simulink model "acc"  (Simulink 7.3)
settings: Solver=ode45  StartTime=0.0  StopTime=1000  RelTol=1e-3
libraries: xbsIndex_r4 x26, xps_library x4, casper_library x4
settings Model: Creator=rprimian  LastModifiedBy=rprimian

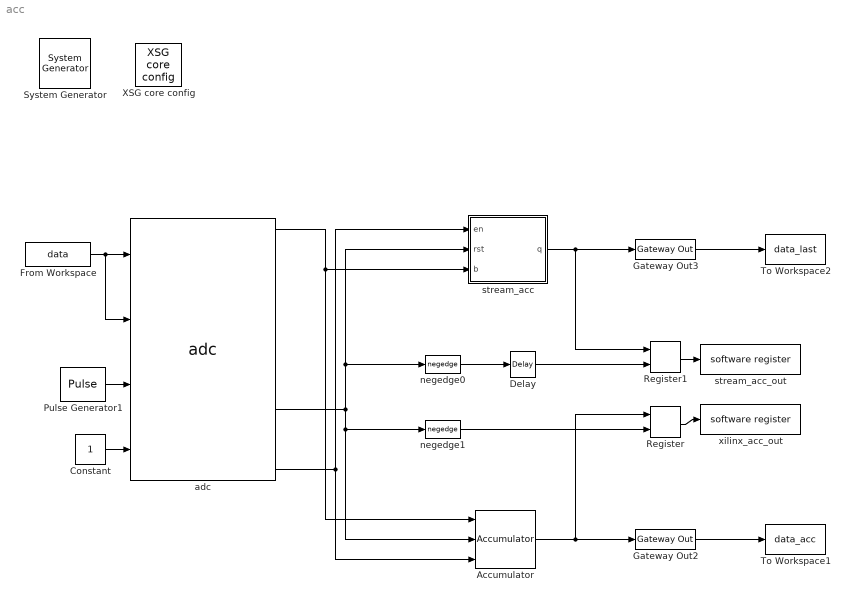
== system acc ==
  " System Generator" : xbsIndex_r4/ System Generator  Tag=genX  SystemSampleTime=-1  xilinxfamily=virtex5  part=xc5vsx95t  speed=-1  package=ff1136  synthesis_tool=XST  clock_wrapper=Clock Enables  directory=./acc/sysgen  testbench=off  simulink_period=1  sysclk_period=3.9062  dcm_input_clock_period=100  incr_netlist=off  trim_vbits=Everywhere in SubSystem  dbl_ovrd=According to Block Masks  core_generation=According to Block Masks  run_coregen=off  deprecated_control=off  eval_field=0  block_type=sysgen
      settings: block_version=11.3
  Accumulator : xbsIndex_r4/Accumulator  operation=Add  n_bits=32  overflow=Flag as error  scale=1  rst=on  hasbypass=off  en=on  dbl_ovrd=off  use_behavioral_HDL=on  implementation=Fabric  block_type=accum
      settings: block_version=11.3
  Constant : Constant  OutDataType=fixdt(1, 16)  OutScaling=2^0
  Delay : xbsIndex_r4/Delay  en=off  latency=7  dbl_ovrd=off  reg_retiming=off  block_type=delay
      settings: block_version=11.3
  From Workspace : FromWorkspace  VariableName=data  SampleTime=0.25  Interpolate=off  OutputAfterFinalValue=Setting to zero
  Gateway Out2 : xbsIndex_r4/Gateway Out  hdl_port=on  timing_constraint=None  locs_specified=off  LOCs={}  block_type=gatewayout
      settings: infoedit="Gateway out block.  Converts Xilinx fixed point inputs into ouputs of type Simulink integer, double, or fixed point.<br><br>Hardware notes:  In hardware these blocks become top level output ports or are discarded, depending on how they are configured."  block_version=11.3
  Gateway Out3 : xbsIndex_r4/Gateway Out  hdl_port=on  timing_constraint=None  locs_specified=off  LOCs={}  block_type=gatewayout
      settings: infoedit="Gateway out block.  Converts Xilinx fixed point inputs into ouputs of type Simulink integer, double, or fixed point.<br><br>Hardware notes:  In hardware these blocks become top level output ports or are discarded, depending on how they are configured."  block_version=11.3
  Pulse Generator1 : DiscretePulseGenerator  Amplitude=1  Period=100  PulseWidth=1  PhaseDelay=50-7  SampleTime=1
  Register : xbsIndex_r4/Register  init=0  rst=off  en=on  dbl_ovrd=off  block_type=register
      settings: block_version=11.3
  Register1 : xbsIndex_r4/Register  init=0  rst=off  en=on  dbl_ovrd=off  block_type=register
      settings: block_version=11.3
  To Workspace1 : ToWorkspace  VariableName=data_acc  SampleTime=-1  SaveFormat=Array
  To Workspace2 : ToWorkspace  VariableName=data_last  SampleTime=-1  SaveFormat=Array
  XSG core config : xps_library/XSG core config  Tag=xps:xsg  SystemSampleTime=-1  hw_sys=ROACH:sx95t  ibob_linux=off  clk_src=adc0_clk  iBOB_clk_src=sys_clk  BEE2_ctrl_clk_src=sys_clk  BEE2_usr_clk_src=sys_clk  ROACH_clk_src=adc0_clk  CORR_clk_src=sys_clk  gpio_clk_io_group=iBOB:sma  gpio_clk_bit_index=0  clk_rate=256  sample_period=1  synthesis_tool=XST  mpc_type=powerpc440_ext
  adc : xps_library/adc  Tag=xps:adc  SystemSampleTime=-1  adc_brd=adc0  adc_clk_rate=1024  adc_interleave=off  sample_period=1
  negedge0 : casper_library/Misc/negedge  Tag=Rising Edge Detector  SystemSampleTime=-1
  negedge1 : casper_library/Misc/negedge  Tag=Rising Edge Detector  SystemSampleTime=-1
  stream_acc : Subsystem  mask{data_type=Signed, bits=32, bin_pt=14, add_latency=2}
      mask prompts: data_type "Output Data Type"; bits "Output Bit Width:"; bin_pt "Output Binary Point:"; add_latency "Adder Latency"
      mask StyleString: popup(Signed|Unsigned),edit,edit,edit
  stream_acc_out : xps_library/software register  Tag=xps:sw_reg  SystemSampleTime=-1  io_dir=To Processor  arith_type=Unsigned  bitwidth=32  bin_pt=0  sample_period=1  gw_name=acc_stream_acc_out_user_data_in
  xilinx_acc_out : xps_library/software register  Tag=xps:sw_reg  SystemSampleTime=-1  io_dir=To Processor  arith_type=Unsigned  bitwidth=32  bin_pt=0  sample_period=1  gw_name=acc_xilinx_acc_out_user_data_in
  wires:
  adc/1 -> Accumulator/1, stream_acc/3(b)
  Accumulator/1 -> Gateway Out2/1, Register/1
  Gateway Out2/1 -> To Workspace1/1
  Gateway Out3/1 -> To Workspace2/1
  stream_acc/1(q) -> Gateway Out3/1, Register1/1
  adc/17 -> stream_acc/1(en), Accumulator/3
  adc/13 -> stream_acc/2(rst), negedge0/1, Accumulator/2, negedge1/1
  From Workspace/1 -> adc/1, adc/2
  Pulse Generator1/1 -> adc/3
  Constant/1 -> adc/4
  Register1/1 -> stream_acc_out/1
  Register/1 -> xilinx_acc_out/1
  negedge0/1 -> Delay/1
  negedge1/1 -> Register/2
  Delay/1 -> Register1/2

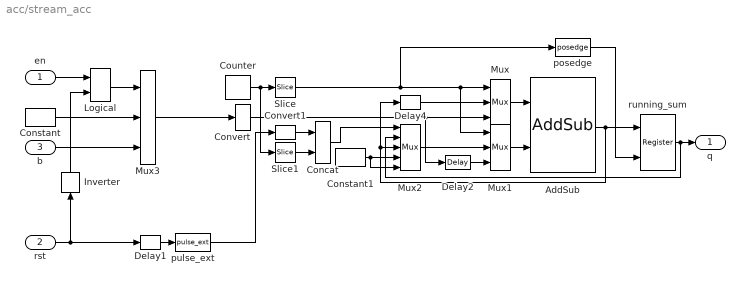
== system acc/stream_acc ==
  en : Inport
  rst : Inport  Port=2
  b : Inport  Port=3
  AddSub : xbsIndex_r4/AddSub  mode=Addition  use_carryin=off  use_carryout=off  en=off  latency=add_latency  precision=User Defined  arith_type="Signed  (2's comp)"  n_bits=32  bin_pt=14  quantization=Truncate  overflow=Flag as error  dbl_ovrd=off  use_behavioral_HDL=off  hw_selection=Fabric  pipelined=off  block_type=addsub
      settings: block_version=11.3
  Concat : xbsIndex_r4/Concat  num_inputs=2  dbl_ovrd=off  block_type=concat
      settings: block_version=11.3
  Constant : xbsIndex_r4/Constant  arith_type=Signed (2's comp)  const=0  n_bits=16  bin_pt=14  explicit_period=on  period=1  equ=P=C  opselect=C  inp2=PCIN>>17  opr=+  inp1=P  carry=CIN  dbl_ovrd=off  block_type=constant
      settings: block_version=11.3
  Constant1 : xbsIndex_r4/Constant  arith_type=Signed (2's comp)  const=0  n_bits=32  bin_pt=14  explicit_period=on  period=1  equ=P=C  opselect=C  inp2=PCIN>>17  opr=+  inp1=P  carry=CIN  dbl_ovrd=off  block_type=constant
      settings: block_version=11.3
  Convert : xbsIndex_r4/Convert  arith_type="Signed  (2's comp)"  n_bits=32  bin_pt=14  quantization=Truncate  overflow=Wrap  latency=0  dbl_ovrd=off  pipeline=off  block_type=convert
      settings: block_version=11.3
  Convert1 : xbsIndex_r4/Convert  arith_type=Unsigned  n_bits=1  bin_pt=0  quantization=Truncate  overflow=Wrap  latency=0  dbl_ovrd=off  pipeline=off  block_type=convert
      settings: block_version=11.3
  Counter : xbsIndex_r4/Counter  cnt_type=Free Running  cnt_to=Inf  operation=Up  start_count=0  cnt_by_val=1  arith_type=Unsigned  n_bits=2  bin_pt=0  load_pin=off  rst=off  en=off  explicit_period=on  period=1  dbl_ovrd=off  use_behavioral_HDL=off  implementation=Fabric  block_type=counter
      settings: block_version=11.3
  Delay1 : xbsIndex_r4/Delay  en=off  latency=7  dbl_ovrd=off  reg_retiming=off  block_type=delay
      settings: block_version=11.3
  Delay2 : xbsIndex_r4/Delay  en=off  latency=2  dbl_ovrd=off  reg_retiming=off  block_type=delay
      settings: block_version=11.3
  Delay4 : xbsIndex_r4/Delay  en=off  latency=1  dbl_ovrd=off  reg_retiming=off  block_type=delay
      settings: block_version=11.3
  Inverter : xbsIndex_r4/Inverter  en=off  latency=0  dbl_ovrd=off  block_type=inv
      settings: block_version=11.3
  Logical : xbsIndex_r4/Logical  logical_function=AND  inputs=2  en=off  latency=0  precision=Full  arith_type=Unsigned  n_bits=16  bin_pt=0  align_bp=on  dbl_ovrd=off  block_type=logical
      settings: block_version=11.3
  Mux : xbsIndex_r4/Mux  inputs=2  en=off  latency=0  precision=Full  arith_type=Unsigned  n_bits=16  bin_pt=14  quantization=Truncate  overflow=Wrap  dbl_ovrd=off  block_type=mux
      settings: block_version=11.3
  Mux1 : xbsIndex_r4/Mux  inputs=2  en=off  latency=0  precision=Full  arith_type=Unsigned  n_bits=16  bin_pt=14  quantization=Truncate  overflow=Wrap  dbl_ovrd=off  block_type=mux
      settings: block_version=11.3
  Mux2 : xbsIndex_r4/Mux  inputs=4  en=off  latency=0  precision=Full  arith_type=Unsigned  n_bits=16  bin_pt=14  quantization=Truncate  overflow=Wrap  dbl_ovrd=off  block_type=mux
      settings: block_version=11.3
  Mux3 : xbsIndex_r4/Mux  inputs=2  en=off  latency=0  precision=Full  arith_type=Unsigned  n_bits=16  bin_pt=14  quantization=Truncate  overflow=Wrap  dbl_ovrd=off  block_type=mux
      settings: block_version=11.3
  Slice : xbsIndex_r4/Slice  nbits=1  boolean_output=on  mode=Upper Bit Location + Width  bit1=0  base1=MSB of Input  bit0=0  base0=LSB of Input  dbl_ovrd=off  block_type=slice
      settings: block_version=11.3
  Slice1 : xbsIndex_r4/Slice  nbits=1  boolean_output=off  mode=Lower Bit Location + Width  bit1=0  base1=MSB of Input  bit0=0  base0=LSB of Input  dbl_ovrd=off  block_type=slice
      settings: block_version=11.3
  posedge : casper_library/Misc/posedge  Tag=Rising Edge Detector  SystemSampleTime=-1
  pulse_ext : casper_library/Misc/pulse_ext  SystemSampleTime=-1  pulse_len=2
  running_sum : xbsIndex_r4/Register  init=0  rst=off  en=on  dbl_ovrd=off  block_type=register
      settings: block_version=11.3
  q : Outport
  wires:
  Mux/1 -> AddSub/1
  Mux1/1 -> AddSub/2
  running_sum/1 -> q/1, Mux2/2
  Convert/1 -> Delay2/1, Mux/3
  Slice/1 -> Mux/1, Mux1/1, posedge/1
  Delay2/1 -> Mux1/3
  Counter/1 -> Slice/1, Slice1/1
  AddSub/1 -> running_sum/1, Delay4/1, Mux2/3
  posedge/1 -> running_sum/2
  Mux2/1 -> Mux1/2
  Delay4/1 -> Mux/2
  Mux3/1 -> Convert/1
  b/1 -> Mux3/3
  Constant/1 -> Mux3/2
  rst/1 -> Inverter/1, Delay1/1
  Constant1/1 -> Mux2/4, Mux2/5
  Logical/1 -> Mux3/1
  en/1 -> Logical/1
  Inverter/1 -> Logical/2
  Delay1/1 -> pulse_ext/1
  pulse_ext/1 -> Convert1/1
  Concat/1 -> Mux2/1
  Convert1/1 -> Concat/1
  Slice1/1 -> Concat/2
